simulink model "modello_simulink"  (R2022b)
settings: Solver=VariableStepAuto  StartTime=0.0  StopTime=40  RelTol=1e-3
values from neighbouring files (symbols this model uses):
  dt = log_vars.dt    [EKF.m]    (also in EKF_for_smoother.m; UKF.m; getJacobian.m; plot_filters.m)
  L = P*H'*inv(S)    [EKF.m]    (also in EKF_for_smoother.m; UKF.m = Pxy*(S)^(-1))
undefined symbols (not defined in the file or in its folder): a, b, IPy, IPz, rp, sigbuilder_block, std_dev_db, std_dev_dx, std_dev_phi_dot, std_dev_psi, std_dev_tau_phi, std_dev_tau_psi, X_start
settings Model: Creator=Giorgia  LastModifiedBy=franc

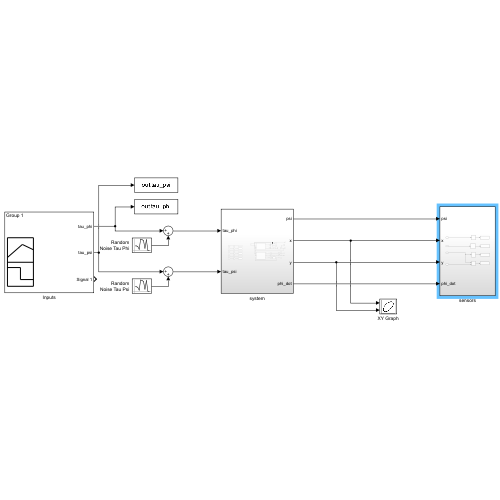
[thumbnail: Simulink's stored preview of the top-level diagram]
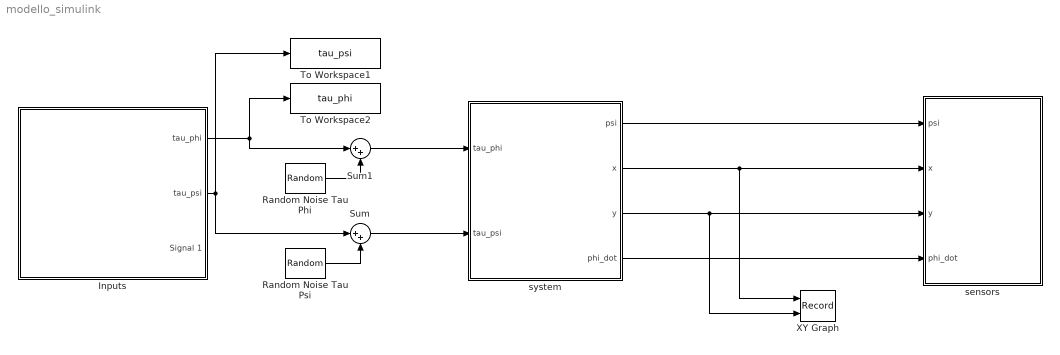
== system modello_simulink ==
  Inputs : Subsystem  Tag=STV Subsys  LoadFcn=sigbuilder_block('load',[5.4 30 1141.2 522.6 ]);  StartFcn=sigbuilder_block('start');  StopFcn=sigbuilder_block('stop');  ClipboardFcn=sigbuilder_block('clipboard');  mask(Sigbuilder block){tuvar=[0:10]}
      mask help: Simulink:masks:SigbuilderBlock_MD
      mask init:
      | if ~strcmp(get_param(bdroot(gcbh),'SimulationStatus'),'stopped') tuvar = sigbuilder_block('maskInit'); end
      settings: CopyFcn=sigbuilder_block('copy');  DeleteFcn=sigbuilder_block('delete');  ModelCloseFcn=sigbuilder_block('modelClose');  PreSaveFcn=sigbuilder_block('preSave');  PauseFcn=sigbuilder_block('pause');  ContinueFcn=sigbuilder_block('continue');  NameChangeFcn=sigbuilder_block('namechange');  OpenFcn=sigbuilder_block('open',[5.4 30 1141.2 522.6 ]);  CloseFcn=sigbuilder_block('close');
      mask Display: plot(0, 0, 100, 100,[2, 2, 32, 32, 2], [68, 8, 8, 68, 68],[32, 2], [38, 38], [32, 19, 2],[53, 60, 44], [32, 17, 17, 2],[16, 16, 31, 31]);txt = getActiveGroup(gcbh);text(2, 100, txt,'verticalAlignment', 'top');
  Random Noise Tau Phi : RandomNumber  Variance=(std_dev_tau_phi)^2  SampleTime=dt
  Random Noise Tau Psi : RandomNumber  Variance=(std_dev_tau_psi)^2  SampleTime=dt
  Sum : Sum  Inputs=|++
  Sum1 : Sum  Inputs=|++
  To Workspace1 : ToWorkspace  VariableName=tau_psi  SampleTime=dt
  To Workspace2 : ToWorkspace  VariableName=tau_phi  SampleTime=dt
  XY Graph : Record  FileSettingsInternal="{\"entries\":[{\"content\":{\"excelSettings\":{\"content\":{},\"type\":\"Streamout.ExcelSettings\"}},\"type\":\"Streamout.FileSettingStorage\",\"uuid\":\"c6e8304d-9aa3-4d04-b47e-ed7e34eded08\"}],\"packageUris\":[\"http://schema.mathworks.com/mf0/streamout_blocks/R2020a\"],\"version\":\"1.0\"}"  Layout=[1 1]  SignalsInternal="{\"entries\":[{\"content\":{\"signals\":[{\"content\":{\"blockPath\":[\"modello_simulink/XY Graph\"],\"channel\":[],\"dimensions\":[1],\"domain\":\"modello_simulink/XY Graph\",\"lineColor\":\"#a2142f\",\"plots\":[1],\"port\":1,\"sid\":[\"\"],\"signalID\":635,\"signalName\":\"system:2\"},\"type\":\"RecordBlkView.Signal\",\"uuid\":\"f08335fb-0b39-4a97-b151-870ade4c6b1b\"},{\"content\":{\"blockPath\":[\"modello_simulink/XY Graph\"],\"channel\":[],\"dimensions\":[1],\"domain\":\"modello_simulink/XY Graph\",\"lineColor\":\"#139fff\",\"plots\":[1],\"port\":2,\"sid\":[\"\"],\"signalID\":639,\"signalName\":\"system:3\"},\"type\":\"RecordBlkView.Signal\",\"uuid\":\"8f7eddf6-a54b-4f66-bef4-9836a0996e7a\"}]},\"type\":\"RecordBlkView.InputSignals\",\"uuid\":\"09ca125a-b73b-494d-bc8d-7a7e0db50771\"}],\"packageUris\":[\"http://schema.mathworks.com/mf0/streamout_blocks/R2020a\"],\"version\":\"1.0\"}"  VisualizationBindings="{\"xyplotplugin\":{\"info\":[{\"series\":[{\"bindingParametersList\":[{\"parameter\":\"X-Axis\",\"signalID\":635,\"signalName\":\"system:2\"},{\"parameter\":\"Y-Axis\",\"signalID\":639,\"signalName\":\"system:3\"}],\"seriesID\":36727}],\"subplotID\":1}]}}"  CompatibilityTag=XY
  sensors : Subsystem
  system : Subsystem
  wires:
  system/1(psi) -> sensors/1(psi)
  system/2(x) -> XY Graph/1, sensors/2(x)
  system/3(y) -> XY Graph/2, sensors/3(y)
  Inputs/2(tau_psi) -> Sum/1, To Workspace1/1
  Sum/1 -> system/2(tau_psi)
  Inputs/1(tau_phi) -> Sum1/1, To Workspace2/1
  Sum1/1 -> system/1(tau_phi)
  system/4(phi_dot) -> sensors/4(phi_dot)
  Random Noise Tau Phi/1 -> Sum1/2
  Random Noise Tau Psi/1 -> Sum/2

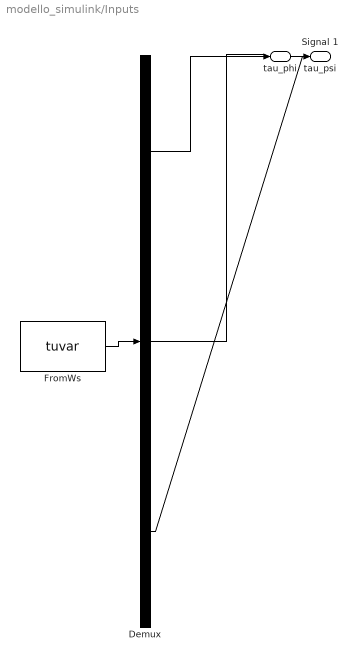
== system modello_simulink/Inputs ==
  Demux : Demux  Tag=STV Demux  Outputs=3
      settings: DisplayOption=none
  FromWs : FromWorkspace  Tag=STV FromWs  VariableName=tuvar
      SigBuilderData=|
      | common.afterFinalStr = 'Extrapolate'
      | common.sampleTime = 0
      | dataSet.timeRange = [0 40]
      | dataSet.name = 'Group 1'
      | sbobj.Groups.Name = 'Group 1'
      | sbobj.Groups.Signals(1).Name = 'tau_phi'
      | sbobj.Groups.Signals(1).XData = [0 25 30 40]
      | sbobj.Groups.Signals(1).YData = [2 2 0 0]
      | sbobj.Groups.Signals(2).Name = 'tau_psi'
      | sbobj.Groups.Signals(2).XData = [0 2 5 6.75 40]
      | sbobj.Groups.Signals(2).YData = [0.5 0.5 0 0 0]
      | sbobj.Groups.Signals(3).Name = 'Signal 1'
      | sbobj.Groups.Signals(3).XData = [0 40]
      | sbobj.Groups.Signals(3).YData = [0 0]
      | sbobj.Groups.TimeRange = [0 40]
  tau_phi : Outport  Tag=STV Outport
  tau_psi : Outport  Tag=STV Outport  Port=2
  Signal 1 : Outport  Tag=STV Outport  Port=3
  wires:
  Demux/1 -> tau_phi/1
  FromWs/1 -> Demux/1
  Demux/2 -> tau_psi/1
  Demux/3 -> Signal 1/1

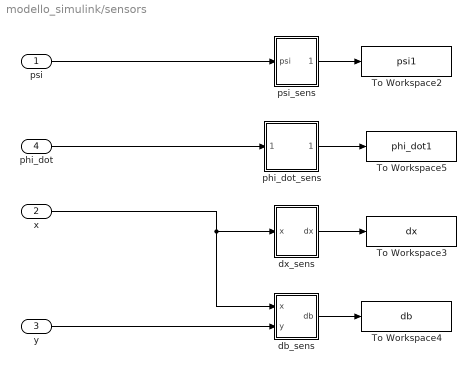
== system modello_simulink/sensors ==
  psi : Inport
  x : Inport  Port=2
  y : Inport  Port=3
  phi_dot : Inport  Port=4
  To Workspace2 : ToWorkspace  VariableName=psi1  SampleTime=dt
  To Workspace3 : ToWorkspace  VariableName=dx  SampleTime=dt
  To Workspace4 : ToWorkspace  VariableName=db  SampleTime=dt
  To Workspace5 : ToWorkspace  VariableName=phi_dot1  SampleTime=dt
  db_sens : Subsystem
  dx_sens : Subsystem
  phi_dot_sens : Subsystem
  psi_sens : Subsystem
  wires:
  x/1 -> db_sens/1(x), dx_sens/1(x)
  psi_sens/1(Output) -> To Workspace2/1
  db_sens/1(db) -> To Workspace4/1
  dx_sens/1(dx) -> To Workspace3/1
  phi_dot_sens/1(Output) -> To Workspace5/1
  psi/1 -> psi_sens/1(psi)
  y/1 -> db_sens/2(y)
  phi_dot/1 -> phi_dot_sens/1(phi_dot)

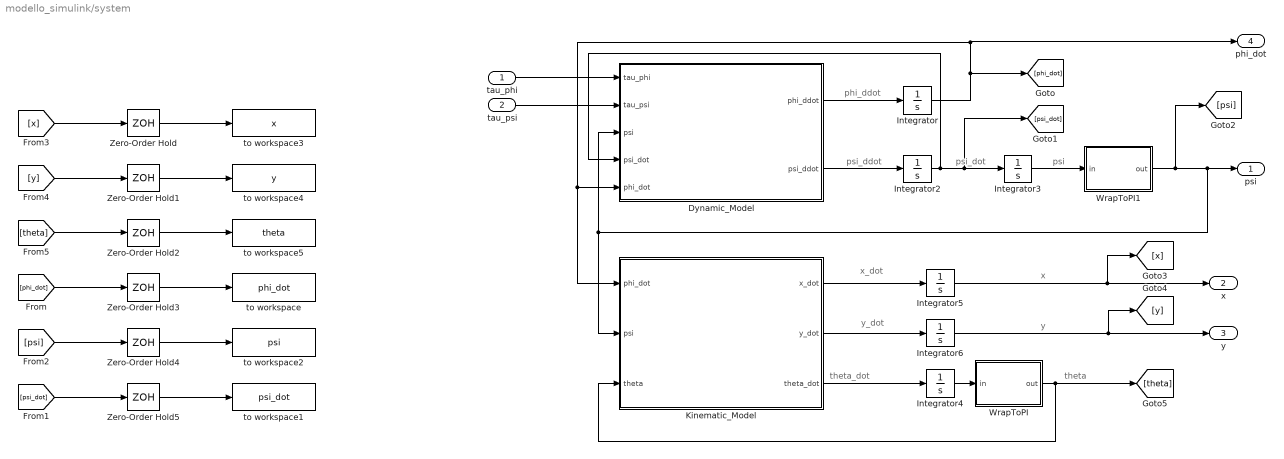
== system modello_simulink/system ==
  note: theta_dot
  note: psi_dot
  note: psi_ddot
  note: phi_ddot
  note: psi
  note: theta
  note: x
  note: x_dot
  note: y
  note: y_dot
  tau_phi : Inport
  tau_psi : Inport  Port=2
  Dynamic_Model : MATLAB Function  TreatAsAtomicUnit=on
  Integrator : Integrator  InitialCondition=X_start(4)
  Integrator2 : Integrator  InitialCondition=X_start(6)
  Integrator3 : Integrator  InitialCondition=X_start(5)
  Integrator4 : Integrator  InitialCondition=X_start(3)
  Integrator5 : Integrator  InitialCondition=X_start(1)
  Integrator6 : Integrator  InitialCondition=X_start(2)
  Kinematic_Model : MATLAB Function  TreatAsAtomicUnit=on
  WrapToPI : MATLAB Function  TreatAsAtomicUnit=on
  WrapToPI1 : MATLAB Function  TreatAsAtomicUnit=on
  Zero-Order Hold{,1..5} (6 alike) : ZeroOrderHold  SampleTime=dt
  to workspace : ToWorkspace  VariableName=phi_dot  SampleTime=dt
  to workspace1 : ToWorkspace  VariableName=psi_dot  SampleTime=dt
  to workspace2 : ToWorkspace  VariableName=psi  SampleTime=dt
  to workspace3 : ToWorkspace  VariableName=x  SampleTime=dt
  to workspace4 : ToWorkspace  VariableName=y  SampleTime=dt
  to workspace5 : ToWorkspace  VariableName=theta  SampleTime=dt
  psi : Outport
  x : Outport  Port=2
  y : Outport  Port=3
  phi_dot : Outport  Port=4
  wires:
  Integrator5/1 -> [x], x/1
  Integrator6/1 -> [y], y/1
  WrapToPI1/1(out) -> [psi], psi/1, Dynamic_Model/3(psi), Kinematic_Model/2(psi)
  Integrator2/1 -> [psi_dot], Integrator3/1, Dynamic_Model/4(psi_dot)
  tau_phi/1 -> Dynamic_Model/1(tau_phi)
  Integrator3/1 -> WrapToPI1/1(in)
  Integrator4/1 -> WrapToPI/1(in)
  tau_psi/1 -> Dynamic_Model/2(tau_psi)
  Integrator/1 -> Kinematic_Model/1(phi_dot), Dynamic_Model/5(phi_dot), phi_dot/1, [phi_dot]
  Kinematic_Model/1(x_dot) -> Integrator5/1
  Kinematic_Model/2(y_dot) -> Integrator6/1
  Kinematic_Model/3(theta_dot) -> Integrator4/1
  Dynamic_Model/2(psi_ddot) -> Integrator2/1
  Dynamic_Model/1(phi_ddot) -> Integrator/1
  WrapToPI/1(out) -> Kinematic_Model/3(theta), [theta]
  [phi_dot] -> Zero-Order Hold3/1
  [psi_dot] -> Zero-Order Hold5/1
  [psi] -> Zero-Order Hold4/1
  [x] -> Zero-Order Hold/1
  [y] -> Zero-Order Hold1/1
  [theta] -> Zero-Order Hold2/1
  Zero-Order Hold/1 -> to workspace3/1
  Zero-Order Hold1/1 -> to workspace4/1
  Zero-Order Hold2/1 -> to workspace5/1
  Zero-Order Hold3/1 -> to workspace/1
  Zero-Order Hold4/1 -> to workspace2/1
  Zero-Order Hold5/1 -> to workspace1/1

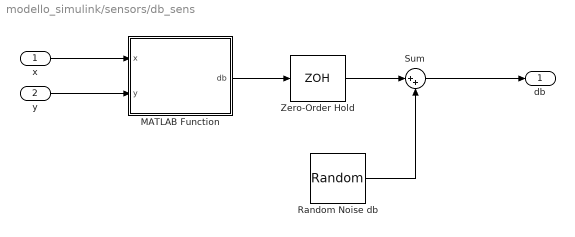
== system modello_simulink/sensors/db_sens ==
  x : Inport
  y : Inport  Port=2
  MATLAB Function : MATLAB Function  TreatAsAtomicUnit=on
  Random Noise db : RandomNumber  Variance=(std_dev_db)^2  SampleTime=dt
  Sum : Sum  Inputs=|++
  Zero-Order Hold : ZeroOrderHold  SampleTime=dt
  db : Outport
  wires:
  MATLAB Function/1(db) -> Zero-Order Hold/1
  y/1 -> MATLAB Function/2(y)
  Zero-Order Hold/1 -> Sum/1
  x/1 -> MATLAB Function/1(x)
  Random Noise db/1 -> Sum/2
  Sum/1 -> db/1

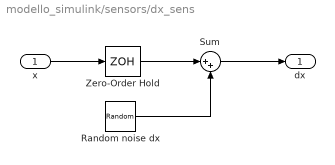
== system modello_simulink/sensors/dx_sens ==
  x : Inport
  Random noise dx : RandomNumber  Variance=(std_dev_dx)^2  SampleTime=dt
  Sum : Sum  Inputs=|++
  Zero-Order Hold : ZeroOrderHold  SampleTime=dt
  dx : Outport
  wires:
  Random noise dx/1 -> Sum/2
  x/1 -> Zero-Order Hold/1
  Zero-Order Hold/1 -> Sum/1
  Sum/1 -> dx/1

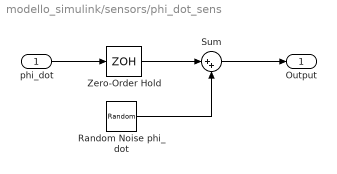
== system modello_simulink/sensors/phi_dot_sens ==
  phi_dot : Inport
  Random Noise phi_dot : RandomNumber  Variance=(std_dev_phi_dot)^2  SampleTime=dt
  Sum : Sum  Inputs=|++
  Zero-Order Hold : ZeroOrderHold  SampleTime=dt
  Output : Outport
  wires:
  Random Noise phi_dot/1 -> Sum/2
  phi_dot/1 -> Zero-Order Hold/1
  Zero-Order Hold/1 -> Sum/1
  Sum/1 -> Output/1

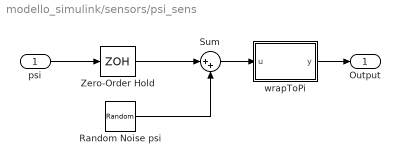
== system modello_simulink/sensors/psi_sens ==
  psi : Inport
  " wrapToPi" : MATLAB Function  TreatAsAtomicUnit=on
  Random Noise psi : RandomNumber  Variance=(std_dev_psi)^2  SampleTime=dt
  Sum : Sum  Inputs=|++
  Zero-Order Hold : ZeroOrderHold  SampleTime=dt
  Output : Outport
  wires:
  Random Noise psi/1 -> Sum/2
  psi/1 -> Zero-Order Hold/1
  Zero-Order Hold/1 -> Sum/1
  Sum/1 -> " wrapToPi"/1(u)
  " wrapToPi"/1(y) -> Output/1

== matlab function modello_simulink/system/Dynamic_Model ==
  data: tau_phi input; phi_ddot output; tau_psi input; psi input; psi_dot input; phi_dot input; psi_ddot output; IPz parameter; IPy parameter; L parameter; rp parameter; b parameter; a parameter
function [phi_ddot,psi_ddot] = DynamicModel(tau_phi,tau_psi,psi,psi_dot,phi_dot,IPz, IPy, L, rp, b, a)
    B = [a*rp^2*cos(psi)^2+b*(rp/L)^2*sin(psi)^2+IPy, -IPz*(rp/L)*sin(psi)
        -IPz*(rp/L)*sin(psi), IPz];
    
    C = [(rp^2*b/L^2-a*rp^2)*cos(psi)*sin(psi)*psi_dot*phi_dot;
            -IPz*rp/L*cos(psi)*psi_dot*phi_dot];

    tau = [tau_phi;
            tau_psi];

    q_ddot = inv(B) * (tau - C);

    phi_ddot = q_ddot(1,:);
    psi_ddot = q_ddot(2,:);

== matlab function modello_simulink/system/Kinematic_Model ==
  data: phi_dot input; x_dot output; psi input; theta input; y_dot output; theta_dot output; rp parameter; L parameter
function [x_dot,y_dot,theta_dot] = KinematicModel(phi_dot,psi,theta,rp, L)
    x_dot = rp * phi_dot * cos(theta) * cos(psi);
    y_dot = rp * phi_dot * sin(theta) * cos(psi);
    theta_dot = - (rp * phi_dot * sin(psi)) / L;

== matlab function modello_simulink/system/WrapToPI ==
  data: in input; out output
function out = wrapper(in)
    out = wrapTo2Pi(in);

== matlab function modello_simulink/system/WrapToPI1 ==
  data: in input; out output
function out = wrapper(in)
    out = wrapToPi(in);

== matlab function modello_simulink/sensors/psi_sens/ wrapToPi ==
  data: u input; y output
function y = fcn(u)
    y = wrapToPi(u);

== matlab function modello_simulink/sensors/db_sens/MATLAB Function ==
  data: x input; db output; y input; D parameter
function db = calculate_db(x,y,D)
db = sqrt(y^2+(D-x)^2);
